simulink model "EV_HPRC_v8_Model"  (R2026a)
settings: Solver=FixedStepAuto  FixedStep=0.01
values from neighbouring files (symbols this model uses):
  g = 9.81    [init_params.m]    (also in run_hprc_v8.m)
  m = 1800    [init_params.m]    (also in run_hprc_v8.m)
  Rw = 0.32    [init_params.m]    (also in run_hprc_v8.m)
libraries: simulink x1
settings Model: Creator=haruc  LastModifiedBy=haruc

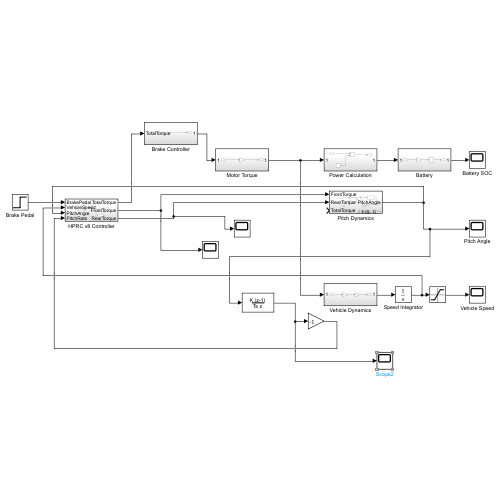
[thumbnail: Simulink's stored preview of the top-level diagram]
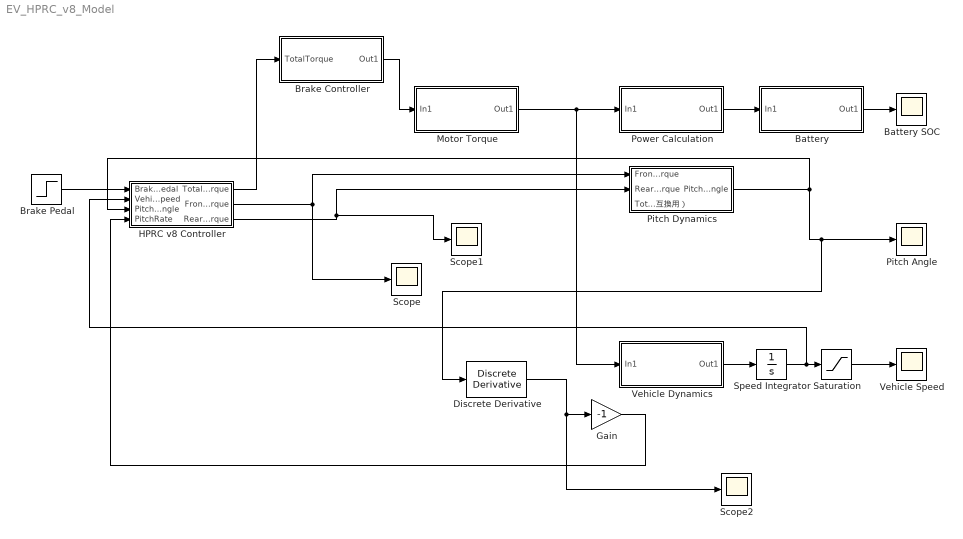
== system EV_HPRC_v8_Model ==
  Battery : Subsystem
  Battery SOC : Scope
      settings: ActiveDisplayYMinimum=-1  ActiveDisplayYMaximum=1
  Brake Controller : Subsystem
  Brake Pedal : Step  SampleTime=0
  Discrete Derivative : simulink/Discrete/Discrete Derivative  gainval=100  ICPrevScaledInput=0.0  OutMin=[]  OutMax=[]  OutDataType=fixdt(1, 16)  OutScaling=2^-10  DoSatur=off
  Gain : Gain  Gain=-1
  HPRC v8 Controller : Subsystem
  Motor Torque : Subsystem
  Pitch Angle : Scope
      settings: ActiveDisplayYMinimum=-0.00010216302147418119  ActiveDisplayYMaximum=0.00091946719326763094  DataLoggingVariableName=ScopeData2
  Pitch Dynamics : Subsystem
  Power Calculation : Subsystem
  Saturation : Saturate  UpperLimit=100  LowerLimit=0
  Scope : Scope
      settings: ActiveDisplayYMinimum=-0.071685532903028953  ActiveDisplayYMaximum=0.64516979612726066  DataLoggingVariableName=ScopeData3
  Scope1 : Scope
      settings: ActiveDisplayYMinimum=-0.054369066833325236  ActiveDisplayYMaximum=0.48932160149992726  DataLoggingVariableName=ScopeData5
  Scope2 : Scope
      settings: ActiveDisplayYMinimum=-0.034566145833333332  ActiveDisplayYMaximum=0.31109531250000005  DataLoggingVariableName=ScopeData8
  Speed Integrator : Integrator  InitialCondition=27.78
  Vehicle Dynamics : Subsystem
  Vehicle Speed : Scope
      settings: ActiveDisplayYMinimum=-3.4724999999999993  ActiveDisplayYMaximum=31.2525
  wires:
  Speed Integrator/1 -> HPRC v8 Controller/2(VehicleSpeed), Saturation/1
  Brake Controller/1(Out1) -> Motor Torque/1(In1)
  Motor Torque/1(Out1) -> Vehicle Dynamics/1(In1), Power Calculation/1(In1)
  Power Calculation/1(Out1) -> Battery/1(In1)
  Battery/1(Out1) -> Battery SOC/1
  Vehicle Dynamics/1(Out1) -> Speed Integrator/1
  Saturation/1 -> Vehicle Speed/1
  Brake Pedal/1 -> HPRC v8 Controller/1(BrakePedal)
  Pitch Dynamics/1(PitchAngle) -> Discrete Derivative/1, Pitch Angle/1, HPRC v8 Controller/3(PitchAngle)
  HPRC v8 Controller/1(TotalTorque) -> Brake Controller/1(TotalTorque)
  HPRC v8 Controller/3(RearTorque) -> Pitch Dynamics/2(RearTorque), Scope1/1
  HPRC v8 Controller/2(FrontTorque) -> Pitch Dynamics/1(FrontTorque), Scope/1
  Gain/1 -> HPRC v8 Controller/4(PitchRate)
  Discrete Derivative/1 -> Scope2/1, Gain/1

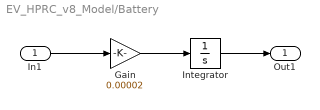
== system EV_HPRC_v8_Model/Battery ==
  In1 : Inport
  Gain : Gain  Gain=0.00002
  Integrator : Integrator  InitialCondition=80
  Out1 : Outport
  wires:
  In1/1 -> Gain/1
  Gain/1 -> Integrator/1
  Integrator/1 -> Out1/1

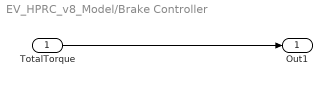
== system EV_HPRC_v8_Model/Brake Controller ==
  TotalTorque : Inport
  Out1 : Outport
  wires:
  TotalTorque/1 -> Out1/1

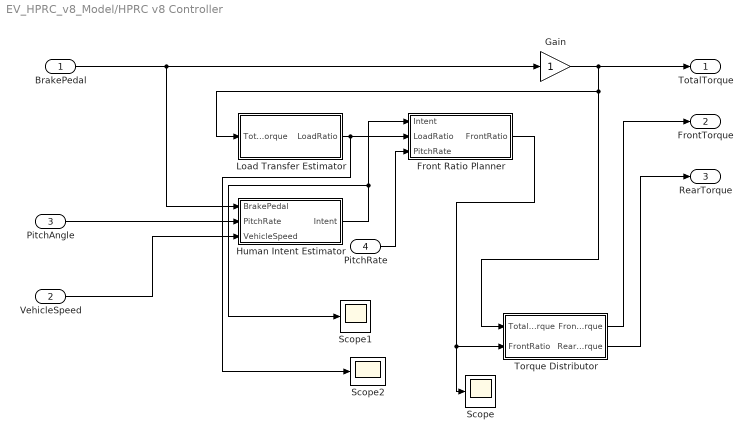
== system EV_HPRC_v8_Model/HPRC v8 Controller ==
  BrakePedal : Inport
  VehicleSpeed : Inport  Port=2
  PitchAngle : Inport  Port=3
  PitchRate : Inport  Port=4
  Front Ratio Planner : Subsystem
  Gain : Gain
  Human Intent Estimator : Subsystem
  Load Transfer Estimator : Subsystem
  Scope : Scope
      settings: ActiveDisplayYMinimum=0.46810941749545282  ActiveDisplayYMaximum=0.6079878425005053  DataLoggingVariableName=ScopeData4
  Scope1 : Scope
      settings: ActiveDisplayYMinimum=0.081249999999999989  ActiveDisplayYMaximum=0.76875  DataLoggingVariableName=ScopeData6
  Scope2 : Scope
      settings: ActiveDisplayYMinimum=-0.010863335416565537  ActiveDisplayYMaximum=0.097770018749089846  DataLoggingVariableName=ScopeData7
  Torque Distributor : Subsystem
  TotalTorque : Outport
  FrontTorque : Outport  Port=2
  RearTorque : Outport  Port=3
  wires:
  BrakePedal/1 -> Gain/1, Human Intent Estimator/1(BrakePedal)
  Gain/1 -> Load Transfer Estimator/1(TotalTorque), Torque Distributor/1(TotalTorque), TotalTorque/1
  VehicleSpeed/1 -> Human Intent Estimator/3(VehicleSpeed)
  PitchAngle/1 -> Human Intent Estimator/2(PitchRate)
  Human Intent Estimator/1(Intent) -> Scope1/1, Front Ratio Planner/1(Intent)
  Load Transfer Estimator/1(LoadRatio) -> Scope2/1, Front Ratio Planner/2("LoadRatio ")
  PitchRate/1 -> Front Ratio Planner/3(PitchRate)
  Front Ratio Planner/1(FrontRatio) -> Scope/1, Torque Distributor/2(FrontRatio)
  Torque Distributor/1(FrontTorque) -> FrontTorque/1
  Torque Distributor/2(RearTorque) -> RearTorque/1

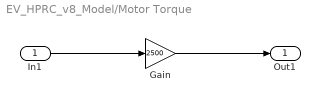
== system EV_HPRC_v8_Model/Motor Torque ==
  In1 : Inport
  Gain : Gain  Gain=2500
  Out1 : Outport
  wires:
  In1/1 -> Gain/1
  Gain/1 -> Out1/1

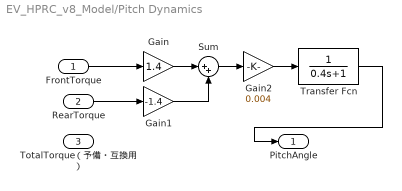
== system EV_HPRC_v8_Model/Pitch Dynamics ==
  FrontTorque : Inport
  RearTorque : Inport  Port=2
  TotalTorque（予備・互換用） : Inport  Port=3
  Gain : Gain  Gain=1.4
  Gain1 : Gain  Gain=-1.4
  Gain2 : Gain  Gain=0.004
  Sum : Sum  Inputs=|++
  Transfer Fcn : TransferFcn  Denominator=[0.4 1]
  PitchAngle : Outport
  wires:
  FrontTorque/1 -> Gain/1
  Gain/1 -> Sum/1
  Transfer Fcn/1 -> PitchAngle/1
  RearTorque/1 -> Gain1/1
  Gain1/1 -> Sum/2
  Sum/1 -> Gain2/1
  Gain2/1 -> Transfer Fcn/1

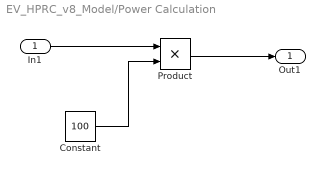
== system EV_HPRC_v8_Model/Power Calculation ==
  In1 : Inport
  Constant : Constant  Value=100
  Product : Product
  Out1 : Outport
  wires:
  In1/1 -> Product/1
  Constant/1 -> Product/2
  Product/1 -> Out1/1

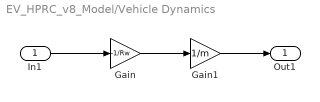
== system EV_HPRC_v8_Model/Vehicle Dynamics ==
  In1 : Inport
  Gain : Gain  Gain=-1/Rw
  Gain1 : Gain  Gain=1/m
  Out1 : Outport
  wires:
  In1/1 -> Gain/1
  Gain1/1 -> Out1/1
  Gain/1 -> Gain1/1

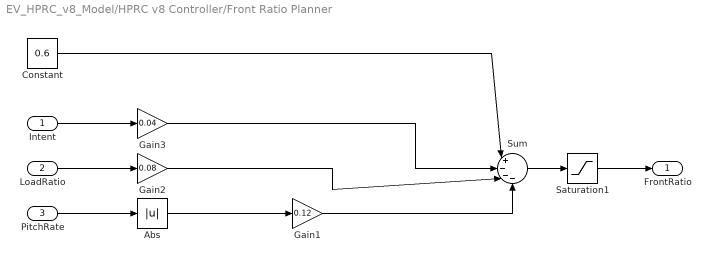
== system EV_HPRC_v8_Model/HPRC v8 Controller/Front Ratio Planner ==
  Intent : Inport
  "LoadRatio " : Inport  Port=2
  PitchRate : Inport  Port=3
  Abs : Abs  SaturateOnIntegerOverflow=off
  Constant : Constant  Value=0.6
  Gain1 : Gain  Gain=0.12
  Gain2 : Gain  Gain=0.08
  Gain3 : Gain  Gain=0.04
  Saturation1 : Saturate  UpperLimit=0.65  LowerLimit=0.35
  Sum : Sum  Inputs=|+---
  FrontRatio : Outport
  wires:
  PitchRate/1 -> Abs/1
  "LoadRatio "/1 -> Gain2/1
  Intent/1 -> Gain3/1
  Saturation1/1 -> FrontRatio/1
  Sum/1 -> Saturation1/1
  Gain2/1 -> Sum/3
  Gain1/1 -> Sum/4
  Gain3/1 -> Sum/2
  Constant/1 -> Sum/1
  Abs/1 -> Gain1/1

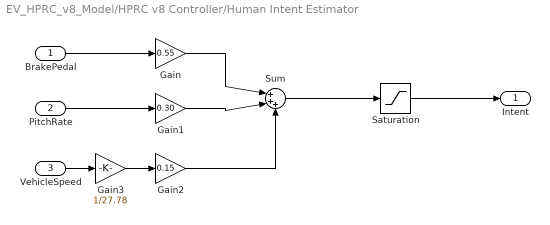
== system EV_HPRC_v8_Model/HPRC v8 Controller/Human Intent Estimator ==
  BrakePedal : Inport
  PitchRate : Inport  Port=2
  VehicleSpeed : Inport  Port=3
  Gain : Gain  Gain=0.55
  Gain1 : Gain  Gain=0.30
  Gain2 : Gain  Gain=0.15
  Gain3 : Gain  Gain=1/27.78
  Saturation : Saturate  UpperLimit=1  LowerLimit=0
  Sum : Sum  Inputs=|+++
  Intent : Outport
  wires:
  Saturation/1 -> Intent/1
  Sum/1 -> Saturation/1
  VehicleSpeed/1 -> Gain3/1
  Gain3/1 -> Gain2/1
  BrakePedal/1 -> Gain/1
  PitchRate/1 -> Gain1/1
  Gain1/1 -> Sum/2
  Gain/1 -> Sum/1
  Gain2/1 -> Sum/3

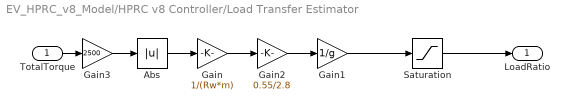
== system EV_HPRC_v8_Model/HPRC v8 Controller/Load Transfer Estimator ==
  TotalTorque : Inport
  Abs : Abs  SaturateOnIntegerOverflow=off
  Gain : Gain  Gain=1/(Rw*m)
  Gain1 : Gain  Gain=1/g
  Gain2 : Gain  Gain=0.55/2.8
  Gain3 : Gain  Gain=2500
  Saturation : Saturate  UpperLimit=0.15  LowerLimit=0
  LoadRatio : Outport
  wires:
  TotalTorque/1 -> Gain3/1
  Abs/1 -> Gain/1
  Gain/1 -> Gain2/1
  Gain2/1 -> Gain1/1
  Gain1/1 -> Saturation/1
  Saturation/1 -> LoadRatio/1
  Gain3/1 -> Abs/1

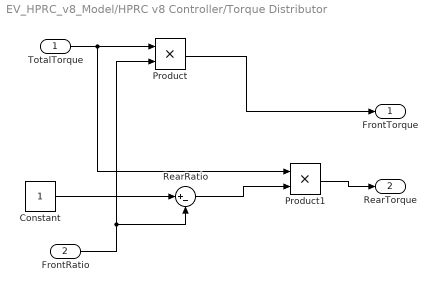
== system EV_HPRC_v8_Model/HPRC v8 Controller/Torque Distributor ==
  TotalTorque : Inport
  FrontRatio : Inport  Port=2
  Constant : Constant
  Product : Product
  Product1 : Product
  RearRatio : Sum  Inputs=|+-
  FrontTorque : Outport
  RearTorque : Outport  Port=2
  wires:
  Constant/1 -> RearRatio/1
  FrontRatio/1 -> RearRatio/2, Product/2
  TotalTorque/1 -> Product1/1, Product/1
  Product/1 -> FrontTorque/1
  RearRatio/1 -> Product1/2
  Product1/1 -> RearTorque/1
